simulink model "simulink_model_casadi_traj_stab"  (R2018a)
settings: Solver=ode4  StartTime=0.0  StopTime=12  FixedStep=12/5000  RelTol=1e-3
undefined symbols (not defined in the file or in its folder): ae1, ae2, at, be, bl, bt, ce, cl, ct, x0
libraries: simulink_extras x3
settings Model: Creator=obrusvit  LastModifiedBy=obrusvit

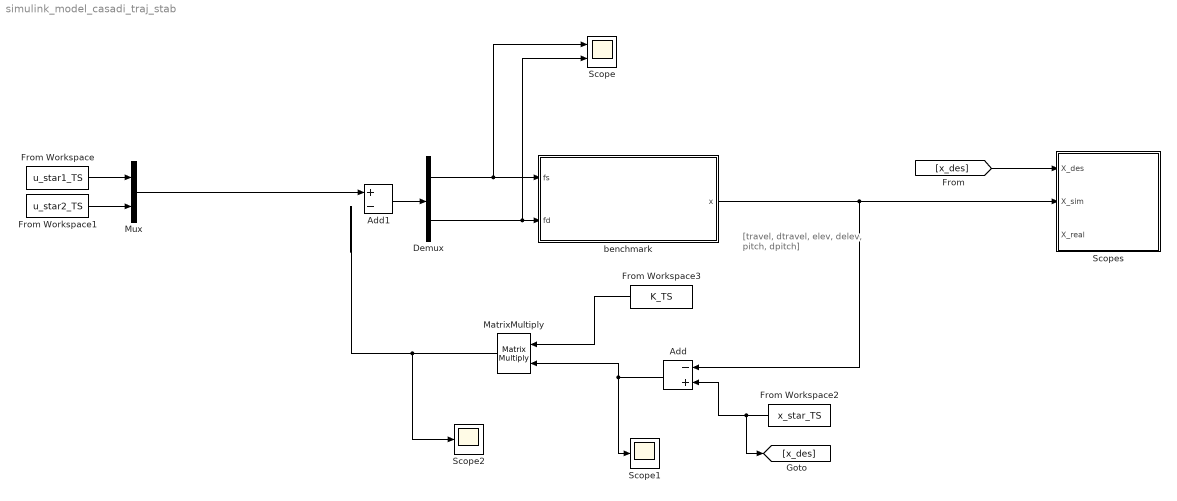
== system simulink_model_casadi_traj_stab ==
  note: [travel, dtravel, elev, delev, pitch, dpitch]
  Add : Sum  Inputs=-+
  Add1 : Sum  Inputs=+-
  Demux : Demux  Outputs=2
  From Workspace : FromWorkspace  VariableName=u_star1_TS  SampleTime=0
  From Workspace1 : FromWorkspace  VariableName=u_star2_TS  SampleTime=0
  From Workspace2 : FromWorkspace  VariableName=x_star_TS  SampleTime=0
  From Workspace3 : FromWorkspace  VariableName=K_TS  SampleTime=0
  MatrixMultiply : Product  Multiplication=Matrix(*)
  Mux : Mux  Inputs=2
  Scope : Scope  NumInputPorts=2
  Scope1 : Scope
  Scope2 : Scope
  Scopes : Subsystem
  benchmark : Subsystem
  wires:
  benchmark/1(x) -> Scopes/2(X_sim), Add/1
  [x_des] -> Scopes/1(X_des)
  Demux/2 -> Scope/2, benchmark/2("fd ")
  Demux/1 -> Scope/1, benchmark/1("fs ")
  Add/1 -> MatrixMultiply/2, Scope1/1
  From Workspace3/1 -> MatrixMultiply/1
  MatrixMultiply/1 -> Scope2/1
  Add1/1 -> Demux/1
  From Workspace1/1 -> Mux/2
  From Workspace/1 -> Mux/1
  From Workspace2/1 -> Add/2, [x_des]
  Mux/1 -> Add1/1

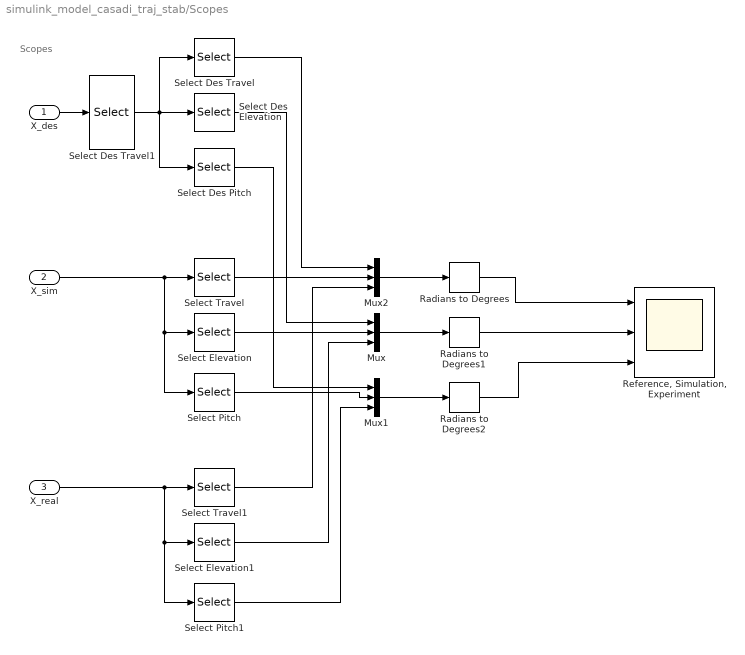
== system simulink_model_casadi_traj_stab/Scopes ==
  note: Scopes
  X_des : Inport
  X_sim : Inport  Port=2
  "X_real " : Inport  Port=3
  Mux : Mux  Inputs=3
  Mux1 : Mux  Inputs=3
  Mux2 : Mux  Inputs=3
  Radians to Degrees : simulink_extras/Transformations/Radians to Degrees
  Radians to Degrees1 : simulink_extras/Transformations/Radians to Degrees
  Radians to Degrees2 : simulink_extras/Transformations/Radians to Degrees
  "Reference, Simulation, Experiment" : Scope  NumInputPorts=3
  Select Des Elevation : Selector  InputPortWidth=3  IndexOptions=Index vector (dialog)  Indices=2  OutputSizes=1
  Select Des Pitch : Selector  InputPortWidth=3  IndexOptions=Index vector (dialog)  Indices=3  OutputSizes=1
  Select Des Travel : Selector  InputPortWidth=3  IndexOptions=Index vector (dialog)  Indices=1  OutputSizes=1
  Select Des Travel1 : Selector  InputPortWidth=6  IndexOptions=Index vector (dialog)  Indices=[1,3,5]  OutputSizes=1
  Select Elevation : Selector  InputPortWidth=6  IndexOptions=Index vector (dialog)  Indices=3  OutputSizes=1
  Select Elevation1 : Selector  InputPortWidth=6  IndexOptions=Index vector (dialog)  Indices=3  OutputSizes=1
  Select Pitch : Selector  InputPortWidth=6  IndexOptions=Index vector (dialog)  Indices=5  OutputSizes=1
  Select Pitch1 : Selector  InputPortWidth=6  IndexOptions=Index vector (dialog)  Indices=5  OutputSizes=1
  Select Travel : Selector  InputPortWidth=6  IndexOptions=Index vector (dialog)  Indices=1  OutputSizes=1
  Select Travel1 : Selector  InputPortWidth=6  IndexOptions=Index vector (dialog)  Indices=1  OutputSizes=1
  wires:
  Mux1/1 -> Radians to Degrees2/1
  X_sim/1 -> Select Pitch/1, Select Elevation/1, Select Travel/1
  Mux2/1 -> Radians to Degrees/1
  Select Elevation/1 -> Mux/2
  Select Pitch/1 -> Mux1/2
  Select Travel/1 -> Mux2/2
  X_des/1 -> Select Des Travel1/1
  Select Des Elevation/1 -> Mux/1
  Select Des Travel/1 -> Mux2/1
  Select Des Pitch/1 -> Mux1/1
  Mux/1 -> Radians to Degrees1/1
  "X_real "/1 -> Select Pitch1/1, Select Elevation1/1, Select Travel1/1
  Select Travel1/1 -> Mux2/3
  Select Elevation1/1 -> Mux/3
  Select Pitch1/1 -> Mux1/3
  Radians to Degrees/1 -> "Reference, Simulation, Experiment"/1
  Radians to Degrees1/1 -> "Reference, Simulation, Experiment"/2
  Radians to Degrees2/1 -> "Reference, Simulation, Experiment"/3
  Select Des Travel1/1 -> Select Des Travel/1, Select Des Pitch/1, Select Des Elevation/1

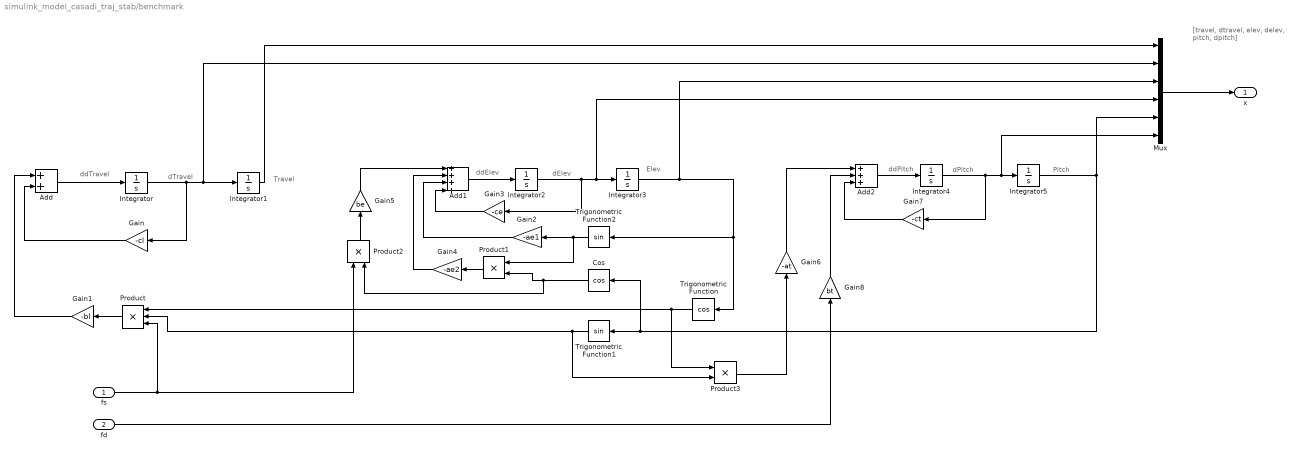
== system simulink_model_casadi_traj_stab/benchmark ==
  note: Pitch
  note: dPitch
  note: ddPitch
  note: Elev
  note: dElev
  note: ddElev
  note: Travel
  note: dTravel
  note: ddTravel
  note: [travel, dtravel, elev, delev, pitch, dpitch]
  "fs " : Inport
  "fd " : Inport  Port=2
  Add : Sum
  Add1 : Sum  Inputs=++++
  Add2 : Sum  Inputs=+++
  Cos : Trigonometry  Operator=cos
  Gain : Gain  Gain=-cl
  Gain1 : Gain  Gain=-bl
  Gain2 : Gain  Gain=-ae1
  Gain3 : Gain  Gain=-ce
  Gain4 : Gain  Gain=-ae2
  Gain5 : Gain  Gain=be
  Gain6 : Gain  Gain=-at
  Gain7 : Gain  Gain=-ct
  Gain8 : Gain  Gain=bt
  Integrator : Integrator  InitialCondition=x0(2)
  Integrator1 : Integrator  InitialCondition=x0(1)
  Integrator2 : Integrator  InitialCondition=x0(4)
  Integrator3 : Integrator  InitialCondition=x0(3)
  Integrator4 : Integrator  InitialCondition=x0(6)
  Integrator5 : Integrator  InitialCondition=x0(5)
  Mux : Mux  Inputs=6
  Product : Product  Inputs=3
  Product1 : Product
  Product2 : Product
  Product3 : Product
  Trigonometric Function : Trigonometry  Operator=cos
  Trigonometric Function1 : Trigonometry
  Trigonometric Function2 : Trigonometry
  x : Outport
  wires:
  Gain5/1 -> Add1/1
  Product/1 -> Gain1/1
  Product2/1 -> Gain5/1
  "fd "/1 -> Gain8/1
  Trigonometric Function/1 -> Product3/1, Product/1
  Product3/1 -> Gain6/1
  Gain7/1 -> Add2/3
  Cos/1 -> Product2/2, Product1/2
  Gain4/1 -> Add1/2
  Gain2/1 -> Add1/3
  Mux/1 -> x/1
  Gain8/1 -> Add2/2
  Add2/1 -> Integrator4/1
  Gain6/1 -> Add2/1
  Integrator1/1 -> Mux/1
  Gain1/1 -> Add/1
  Integrator3/1 -> Mux/3, Trigonometric Function2/1, Trigonometric Function/1
  Integrator2/1 -> Gain3/1, Mux/4, Integrator3/1
  Product1/1 -> Gain4/1
  Gain3/1 -> Add1/4
  Integrator4/1 -> Gain7/1, Mux/6, Integrator5/1
  Integrator/1 -> Gain/1, Mux/2, Integrator1/1
  Gain/1 -> Add/2
  Add1/1 -> Integrator2/1
  Integrator5/1 -> Mux/5, Cos/1, Trigonometric Function1/1
  Trigonometric Function2/1 -> Product1/1, Gain2/1
  Trigonometric Function1/1 -> Product3/2, Product/2
  "fs "/1 -> Product2/1, Product/3
  Add/1 -> Integrator/1
